simulink model "wave"  (R2017a)
settings: Solver=VariableStepAuto  StartTime=0.0  StopTime=10.0  RelTol=1e-3
libraries: commsynccomp2 x2, dspmathops x1
settings Model: Creator=carvalho  LastModifiedBy=carvalho

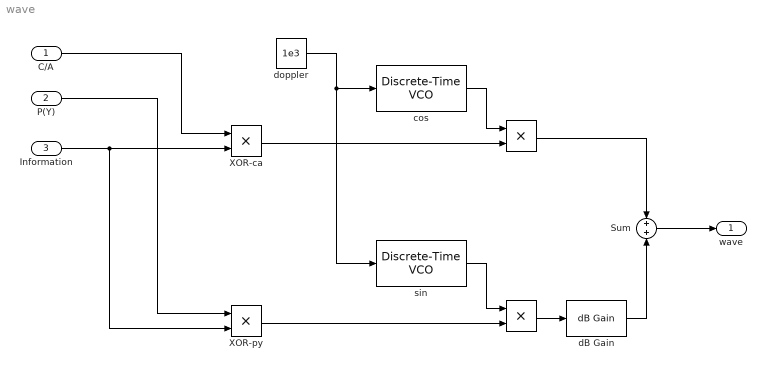
== system wave ==
  C/A : Inport
  P(Y) : Inport  Port=2
  Information : Inport  Port=3
  " " : Product
  " " : Product
  Sum : Sum  Inputs=+|+
  XOR-ca : Product
  XOR-py : Product
  "cos " : commsynccomp2/Discrete-Time VCO  Ac=1  Fc=4.092e6  Kc=1  Ph=0  ts=1/(16.368e6)
      settings: SourceProductName=Communications System Toolbox  SourceProductBaseCode=CM
  dB Gain : dspmathops/dB Gain  dB=-3  intype=Amplitude
      settings: SourceProductName=DSP System Toolbox  SourceProductBaseCode=DS
  doppler : Constant  Value=1e3
  "sin " : commsynccomp2/Discrete-Time VCO  Ac=1  Fc=4.092e6  Kc=1  Ph=1.5708  ts=1/(16.368e6)
      settings: SourceProductName=Communications System Toolbox  SourceProductBaseCode=CM
  wave : Outport
  wires:
  XOR-py/1 -> " "/2
  XOR-ca/1 -> " "/2
  " "/1 -> Sum/1
  "sin "/1 -> " "/1
  " "/1 -> dB Gain/1
  "cos "/1 -> " "/1
  doppler/1 -> "sin "/1, "cos "/1
  dB Gain/1 -> Sum/2
  Sum/1 -> wave/1
  C/A/1 -> XOR-ca/1
  P(Y)/1 -> XOR-py/1
  Information/1 -> XOR-py/2, XOR-ca/2
